simulink model "DUC"  (R2022a)
settings: Solver=VariableStepAuto  StartTime=0.0  StopTime=sample_period*512*300  RelTol=1e-3
InitFcn:
  | sample_period=1/400e6;
  | coeffs_AIE_scaling;
  | dds=75e6; % ddfs frequency
undefined symbols (not defined in the file or in its folder): None, S, vsva2197, xcvc1902
libraries: aieDSP x10, aieBasic x4, dspmlti4 x4, aieUtilities x2, vmcUtilities x1
settings Model: Creator=mmi  LastModifiedBy=robg
settings DebuggingCC: ParameterOverflowMsg=warning  UnconnectedInputMsg=warning  UnconnectedOutputMsg=warning  UnconnectedLineMsg=warning
settings HardwareCC: ProdBitPerPointer=32  ProdBitPerSizeT=32  ProdBitPerPtrDiffT=32  ProdLargestAtomicFloat=None  ProdIntDivRoundTo=Undefined  ProdEndianess=Unspecified  ProdWordSize=32  ProdHWDeviceType=ASIC/FPGA->ASIC/FPGA  TargetBitPerLong=64  TargetBitPerPointer=64  TargetBitPerSizeT=64  TargetBitPerPtrDiffT=64  TargetLongLongMode=on  TargetIntDivRoundTo=Zero  TargetEndianess=LittleEndian  TargetWordSize=64  TargetHWDeviceType=Custom Processor->MATLAB Host Computer  ProdEqTarget=off
settings RTWCC: DLArmComputeVersion=19.05

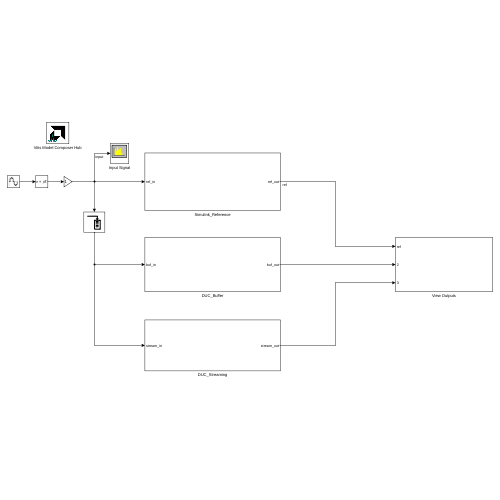
[thumbnail: Simulink's stored preview of the top-level diagram]
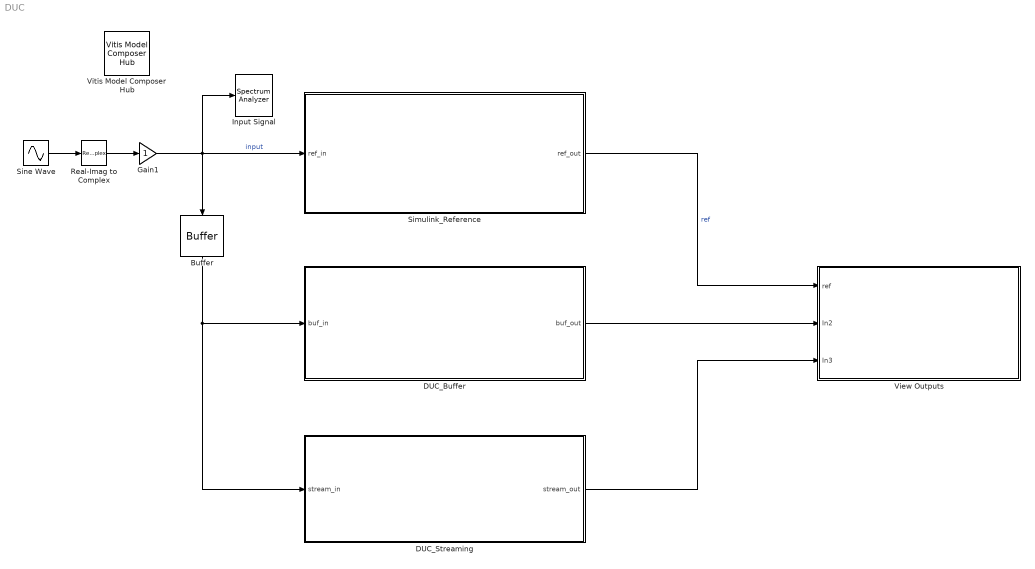
== system DUC ==
  Buffer : Buffer  N=32  OutputFrames=off
  DUC_Buffer : Subsystem
  DUC_Streaming : Subsystem
  Gain1 : Gain  OutDataTypeStr=fixdt(1,32,0)  RndMeth=Convergent
  Input Signal : SpectrumAnalyzer  DefaultConfigurationName=spbscopes.SpectrumAnalyzerBlockCfg
  Real-Imag to Complex : RealImagToComplex  Input=Real
  Simulink_Reference : Subsystem
  Sine Wave : Sin  Amplitude=1000  Frequency=2*pi*1e6  SampleTime=16*sample_period
  View Outputs : Subsystem
  Vitis Model Composer Hub : vmcUtilities/Vitis Model Composer Hub  Tag=genX  CodeGeneration=off  SubsystemName=DUC_Streaming  CompilationType=AIECompilation  ExportTypeV2=Graph Code  TargetDirectory=./duc_strm  exportDesign=off  analyzeDesign=on  validateDesignOnHw=off  ExportType=AI Engines  IpVendor=xilinx.com  IpLibrary=hls  IpVersion=1.0  IpHWLanguage=Verilog  AieCompilerOptions={}  AieSimulatorOptions={}  CreateTestbench=on  TestbenchStackSize=10  RunRtlSim=off  RunCSim=off  RunAieSim=on  AieSimTimeout=50000  RunAieSimProfiling=off  LaunchVitisAnalyzer=on  PlotOutput=off  RunX86Sim=off  X86SimTimeout=10  GenHwImage=off  GenLibadfXo=off  GenHwValidationCode=off  PlatformType=Not Specified  HwSystemType=Baremetal  HwValidationTarget=hw  ProjDevice=Versal VCK190 Evaluation Platform with New SD Level Shifter (xcvc1902-vsva2197-2MP-e-S)  ProjDevicePart=xcvc1902-vsva2197-2MP-e-S  AIEType=AIE  SamplePeriod=-1  ClockFrequency=200  DataPathParallelism=1  xilinxfamily=versalaicore  part=xcvc1902  speed=-2MP-e-S  package=vsva2197  directory=./netlist  testbench=off  incr_netlist=off  synthesis_tool=Vivado  clock_wrapper=Clock Enables  dbl_ovrd=According to Block Masks  dcm_input_clock_period=10  sysclk_period=sample_period  simulink_period=sample_period  eval_field=0  IPInfoJsonString="{\"AIESubsystem\":{\"SubsystemName\":\"DUC_Streaming\",\"TargetDirectory\":\"./duc_strm\",\"SubsystemDir\":\"./duc_strm/ip/DUC_Streaming\"},\"SubsystemTag\":\"AIENode\"}"  LogFileName=/group/xcoswmktg2/robg/git/vmc_examples/Vitis_Model_Composer/Examples/AIENGINE/DSPlib/DUC/duc_strm/model_composer.log  NThreads=4
  wires:
  Buffer/1 -> DUC_Streaming/1(stream_in), DUC_Buffer/1(buf_in)
  Sine Wave/1 -> Real-Imag to Complex/1
  Real-Imag to Complex/1 -> Gain1/1
  Gain1/1 -> Buffer/1, Input Signal/1, Simulink_Reference/1(ref_in)  "input"
  Simulink_Reference/1(ref_out) -> View Outputs/1(ref)  "ref"
  DUC_Buffer/1(buf_out) -> View Outputs/2(In2)
  DUC_Streaming/1(stream_out) -> View Outputs/3(In3)

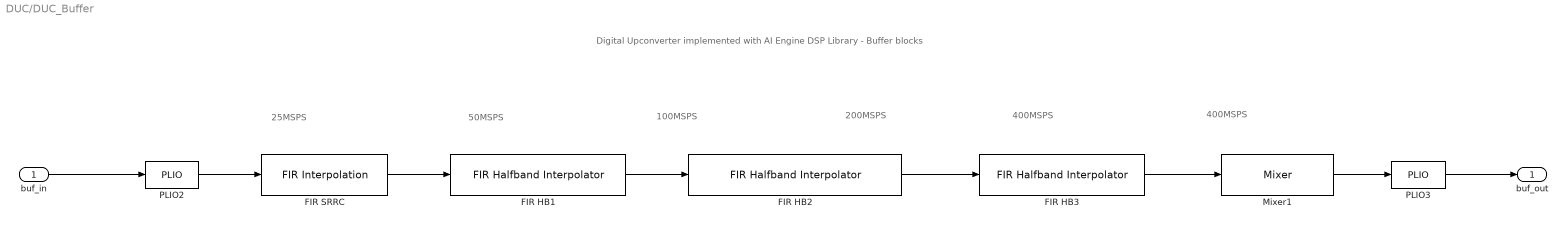
== system DUC/DUC_Buffer ==
  note: Digital Upconverter implemented with AI Engine DSP Library - Buffer blocks
  note: 25MSPS
  note: 400MSPS
  note: 100MSPS
  note: 400MSPS
  note: 50MSPS
  note: 200MSPS
  buf_in : Inport
  FIR HB1 : aieDSP/FIR Halfband Interpolator  data_type=cint32  coef_type=int32  use_coeff_reload=off  dual_ip=off  num_outputs=off  coeff=hb1_dsplib_coeff  fir_length=31  input_window_size=64  shift_val=17  rnd_mode=Round convergent to even  sat_mode=0-None  interp_poly=1  upshift_ct=0  casc_length=1  AIE_VARIANT=1  blockJsonConstraints=[]  blockJsonConstraintsInternal="{\"type\":\"constraint\",\"constraintType\":\"coreUtilization\",\"sid\":\"347:filter.m_firKernels[0]\",\"lhs\":{\"type\":\"runtimeRatio\",\"args\":{\"type\":\"kernel\",\"name\":\"dsplibDUC/AIE_DUC_Win/FIR HB1\",\"sid\":\"347:filter.m_firKernels[0]\"}},\"rhs\":{\"type\":\"evaluable\",\"expr\":\"0.2732\",\"value\":0.2732},\"equality\":true}"  spec=vmc_fir_interpolate_hb.json  SerializedMaskParamNames=[]  SerializedMaskParamValues=[]  SerializedMaskParamVisibilities=[]  block_type=FIR Halfband Interpolator  SerializedMaskParamDataypes=typename|typename|bool|bool|bool|coef_type|uint|uint|uint|uint|uint|uint|uint|uint|uint  SerializedMaskParamEnumStrArr=0|0|0|0|0|0|0|0|0|Floor,Ceiling,Round to positive infinity,Round to negative infinity,Round symmetrical to infinity,Round symmetrical to zero,Round convergent to even,Round convergent to odd|0-None,1-Asymmetric,3-Symmetric|0|0|0|0  SerializedMaskParamEnumValArr=0|0|0|0|0|0|0|0|0|0,1,2,3,4,5,6,7|0,1,3|0|0|0|0  SerializedMaskParamVectorArr=0|0|0|0|0|1|0|0|0|0|0|0|0|0|0
  FIR HB2 : aieDSP/FIR Halfband Interpolator  data_type=cint32  coef_type=int32  use_coeff_reload=off  dual_ip=off  num_outputs=off  coeff=hb2_dsplib_coeff  fir_length=31  input_window_size=128  shift_val=18  rnd_mode=Round convergent to even  sat_mode=0-None  interp_poly=1  upshift_ct=0  casc_length=1  AIE_VARIANT=1  blockJsonConstraints=[]  blockJsonConstraintsInternal="{\"type\":\"constraint\",\"constraintType\":\"coreUtilization\",\"sid\":\"348:filter.m_firKernels[0]\",\"lhs\":{\"type\":\"runtimeRatio\",\"args\":{\"type\":\"kernel\",\"name\":\"dsplibDUC/AIE_DUC_Win/FIR HB2\",\"sid\":\"348:filter.m_firKernels[0]\"}},\"rhs\":{\"type\":\"evaluable\",\"expr\":\"0.4057\",\"value\":0.4057},\"equality\":true}"  spec=vmc_fir_interpolate_hb.json  SerializedMaskParamNames=[]  SerializedMaskParamValues=[]  SerializedMaskParamVisibilities=[]  block_type=FIR Halfband Interpolator  SerializedMaskParamDataypes=typename|typename|bool|bool|bool|coef_type|uint|uint|uint|uint|uint|uint|uint|uint|uint  SerializedMaskParamEnumStrArr=0|0|0|0|0|0|0|0|0|Floor,Ceiling,Round to positive infinity,Round to negative infinity,Round symmetrical to infinity,Round symmetrical to zero,Round convergent to even,Round convergent to odd|0-None,1-Asymmetric,3-Symmetric|0|0|0|0  SerializedMaskParamEnumValArr=0|0|0|0|0|0|0|0|0|0,1,2,3,4,5,6,7|0,1,3|0|0|0|0  SerializedMaskParamVectorArr=0|0|0|0|0|1|0|0|0|0|0|0|0|0|0
  FIR HB3 : aieDSP/FIR Halfband Interpolator  data_type=cint32  coef_type=int32  use_coeff_reload=off  dual_ip=off  num_outputs=off  coeff=hb3_dsplib_coeff  fir_length=31  input_window_size=256  shift_val=16  rnd_mode=Round convergent to even  sat_mode=0-None  interp_poly=1  upshift_ct=0  casc_length=1  AIE_VARIANT=1  blockJsonConstraints=[]  blockJsonConstraintsInternal="{\"type\":\"constraint\",\"constraintType\":\"coreUtilization\",\"sid\":\"349:filter.m_firKernels[0]\",\"lhs\":{\"type\":\"runtimeRatio\",\"args\":{\"type\":\"kernel\",\"name\":\"dsplibDUC/AIE_DUC_Win/FIR HB3\",\"sid\":\"349:filter.m_firKernels[0]\"}},\"rhs\":{\"type\":\"evaluable\",\"expr\":\"0.8048\",\"value\":0.8048},\"equality\":true}"  spec=vmc_fir_interpolate_hb.json  SerializedMaskParamNames=[]  SerializedMaskParamValues=[]  SerializedMaskParamVisibilities=[]  block_type=FIR Halfband Interpolator  SerializedMaskParamDataypes=typename|typename|bool|bool|bool|coef_type|uint|uint|uint|uint|uint|uint|uint|uint|uint  SerializedMaskParamEnumStrArr=0|0|0|0|0|0|0|0|0|Floor,Ceiling,Round to positive infinity,Round to negative infinity,Round symmetrical to infinity,Round symmetrical to zero,Round convergent to even,Round convergent to odd|0-None,1-Asymmetric,3-Symmetric|0|0|0|0  SerializedMaskParamEnumValArr=0|0|0|0|0|0|0|0|0|0,1,2,3,4,5,6,7|0,1,3|0|0|0|0  SerializedMaskParamVectorArr=0|0|0|0|0|1|0|0|0|0|0|0|0|0|0
  FIR SRRC : aieDSP/FIR Interpolation  data_type=cint32  coef_type=int32  use_coeff_reload=off  num_outputs=off  coeff=srrc_coeff  fir_length=32  interpolate_factor=2  input_window_size=32  shift_val=12  rnd_mode=Round convergent to even  sat_mode=0-None  interp_poly=1  casc_length=1  AIE_VARIANT=1  blockJsonConstraints=[]  blockJsonConstraintsInternal="{\"type\":\"constraint\",\"constraintType\":\"coreUtilization\",\"sid\":\"350:filter.m_firKernels[0]\",\"lhs\":{\"type\":\"runtimeRatio\",\"args\":{\"type\":\"kernel\",\"name\":\"dsplibDUC/AIE_DUC_Win/FIR SRRC\",\"sid\":\"350:filter.m_firKernels[0]\"}},\"rhs\":{\"type\":\"evaluable\",\"expr\":\"0.5155\",\"value\":0.5155},\"equality\":true}"  spec=vmc_fir_interpolate_asym.json  SerializedMaskParamNames=[]  SerializedMaskParamValues=[]  SerializedMaskParamVisibilities=[]  block_type=FIR Interpolation  SerializedMaskParamDataypes=typename|typename|bool|bool|coef_type|uint|uint|uint|uint|uint|uint|uint|uint|uint  SerializedMaskParamEnumStrArr=0|0|0|0|0|0|0|0|0|Floor,Ceiling,Round to positive infinity,Round to negative infinity,Round symmetrical to infinity,Round symmetrical to zero,Round convergent to even,Round convergent to odd|0-None,1-Asymmetric,3-Symmetric|0|0|0  SerializedMaskParamEnumValArr=0|0|0|0|0|0|0|0|0|0,1,2,3,4,5,6,7|0,1,3|0|0|0  SerializedMaskParamVectorArr=0|0|0|0|1|0|0|0|0|0|0|0|0|0
  Mixer1 : aieDSP/Mixer  data_type=cint32  input_window_size=512  rnd_mode=Round to positive infinity  sat_mode=0-None  mixer_mode=Single Input Mode  USE_PHASE_RELOAD=off  phase_increment=805306368 % 75*2^32/400  AIE_VARIANT=1  blockJsonConstraints=[]  blockJsonConstraintsInternal=[]  spec=vmc_mixer.json  SerializedMaskParamNames=[]  SerializedMaskParamValues=[]  SerializedMaskParamVisibilities=[]  block_type=Mixer  SerializedMaskParamDataypes=typename|uint|uint|uint|uint|bool|uint|uint  SerializedMaskParamEnumStrArr=0|0|Floor,Ceiling,Round to positive infinity,Round to negative infinity,Round symmetrical to infinity,Round symmetrical to zero,Round convergent to even,Round convergent to odd|0-None,1-Asymmetric,3-Symmetric|Single Input Mode,Dual Input Mode|0|0|0  SerializedMaskParamEnumValArr=0|0|0,1,2,3,4,5,6,7|0,1,3|1,2|0|0|0  SerializedMaskParamVectorArr=0|0|0|0|0|0|0|0
  PLIO2 : aieBasic/PLIO  PlioWidth=64  PlioFreqSpec=on  PlioFreq=500  ColLocation=0  channel=0  blockJsonConstraints=[]  deprecateConstraints=0
  PLIO3 : aieBasic/PLIO  PlioWidth=64  PlioFreqSpec=on  PlioFreq=500  ColLocation=0  channel=0  blockJsonConstraints=[]  deprecateConstraints=0
  buf_out : Outport
  wires:
  PLIO2/1 -> FIR SRRC/1
  FIR HB1/1 -> FIR HB2/1
  FIR HB2/1 -> FIR HB3/1
  buf_in/1 -> PLIO2/1
  PLIO3/1 -> buf_out/1
  FIR HB3/1 -> Mixer1/1
  FIR SRRC/1 -> FIR HB1/1
  Mixer1/1 -> PLIO3/1

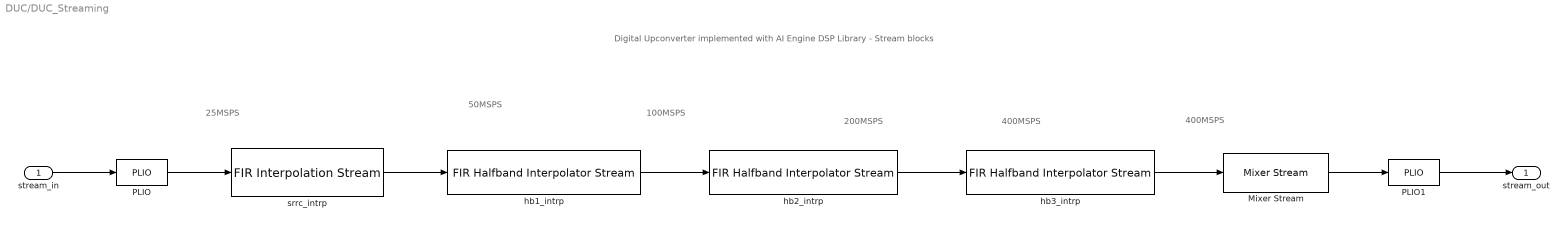
== system DUC/DUC_Streaming ==
  note: Digital Upconverter implemented with AI Engine DSP Library - Stream blocks
  note: 25MSPS
  note: 50MSPS
  note: 100MSPS
  note: 200MSPS
  note: 400MSPS
  note: 400MSPS
  stream_in : Inport
  Mixer Stream : aieDSP/Mixer Stream  data_type=cint32  input_window_size=512  mixer_mode=Single Input Mode  ssr=1  rnd_mode=Round to positive infinity  sat_mode=0-None  phase_increment=805306368 % 75*2^32/400  USE_PHASE_RELOAD=off  initial_phase_offset=0  AIE_VARIANT=1  blockJsonConstraints=[]  blockJsonConstraintsInternal=[]  spec=vmc_stream_mixer.json  SerializedMaskParamNames=[]  SerializedMaskParamValues=[]  SerializedMaskParamVisibilities=[]  block_type=Mixer Stream  SerializedMaskParamDataypes=typename|uint|uint|uint|uint|uint|uint|bool|uint|uint  SerializedMaskParamEnumStrArr=0|0|Single Input Mode,Dual Input Mode|0|Floor,Ceiling,Round to positive infinity,Round to negative infinity,Round symmetrical to infinity,Round symmetrical to zero,Round convergent to even,Round convergent to odd|0-None,1-Asymmetric,3-Symmetric|0|0|0|0  SerializedMaskParamEnumValArr=0|0|1,2|0|0,1,2,3,4,5,6,7|0,1,3|0|0|0|0  SerializedMaskParamVectorArr=0|0|0|0|0|0|0|0|0|0
  PLIO : aieBasic/PLIO  PlioWidth=64  PlioFreqSpec=on  PlioFreq=250  ColLocation=0  channel=0  blockJsonConstraints=[]  deprecateConstraints=0
  PLIO1 : aieBasic/PLIO  PlioWidth=64  PlioFreqSpec=on  PlioFreq=500  ColLocation=0  channel=0  blockJsonConstraints=[]  deprecateConstraints=0
  hb1_intrp : aieDSP/FIR Halfband Interpolator Stream  data_type=cint32  coef_type=int32  use_coeff_reload=off  dual_ip=off  num_outputs=off  coeff=hb1_dsplib_coeff  fir_length=31  input_window_size=64  shift_val=17  rnd_mode=Round convergent to even  sat_mode=0-None  ssr=1  interp_poly=1  upshift_ct=0  casc_length=2  AIE_VARIANT=1  blockJsonConstraints=[]  blockJsonConstraintsInternal=[]  spec=vmc_stream_fir_interpolate_hb.json  SerializedMaskParamNames=[]  SerializedMaskParamValues=[]  SerializedMaskParamVisibilities=[]  block_type=FIR Halfband Interpolator Stream  SerializedMaskParamDataypes=typename|typename|bool|bool|bool|coef_type|uint|uint|uint|uint|uint|uint|uint|uint|uint|uint  SerializedMaskParamEnumStrArr=0|0|0|0|0|0|0|0|0|Floor,Ceiling,Round to positive infinity,Round to negative infinity,Round symmetrical to infinity,Round symmetrical to zero,Round convergent to even,Round convergent to odd|0-None,1-Asymmetric,3-Symmetric|0|0|0|0|0  SerializedMaskParamEnumValArr=0|0|0|0|0|0|0|0|0|0,1,2,3,4,5,6,7|0,1,3|0|0|0|0|0  SerializedMaskParamVectorArr=0|0|0|0|0|1|0|0|0|0|0|0|0|0|0|0
  hb2_intrp : aieDSP/FIR Halfband Interpolator Stream  data_type=cint32  coef_type=int32  use_coeff_reload=off  dual_ip=off  num_outputs=off  coeff=hb2_dsplib_coeff  fir_length=31  input_window_size=128  shift_val=18  rnd_mode=Round convergent to even  sat_mode=0-None  ssr=1  interp_poly=1  upshift_ct=0  casc_length=1  AIE_VARIANT=1  blockJsonConstraints=[]  blockJsonConstraintsInternal=[]  spec=vmc_stream_fir_interpolate_hb.json  SerializedMaskParamNames=[]  SerializedMaskParamValues=[]  SerializedMaskParamVisibilities=[]  block_type=FIR Halfband Interpolator Stream  SerializedMaskParamDataypes=typename|typename|bool|bool|bool|coef_type|uint|uint|uint|uint|uint|uint|uint|uint|uint|uint  SerializedMaskParamEnumStrArr=0|0|0|0|0|0|0|0|0|Floor,Ceiling,Round to positive infinity,Round to negative infinity,Round symmetrical to infinity,Round symmetrical to zero,Round convergent to even,Round convergent to odd|0-None,1-Asymmetric,3-Symmetric|0|0|0|0|0  SerializedMaskParamEnumValArr=0|0|0|0|0|0|0|0|0|0,1,2,3,4,5,6,7|0,1,3|0|0|0|0|0  SerializedMaskParamVectorArr=0|0|0|0|0|1|0|0|0|0|0|0|0|0|0|0
  hb3_intrp : aieDSP/FIR Halfband Interpolator Stream  data_type=cint32  coef_type=int32  use_coeff_reload=off  dual_ip=off  num_outputs=off  coeff=hb3_dsplib_coeff  fir_length=31  input_window_size=256  shift_val=16  rnd_mode=Round convergent to even  sat_mode=0-None  ssr=1  interp_poly=1  upshift_ct=0  casc_length=1  AIE_VARIANT=1  blockJsonConstraints=[]  blockJsonConstraintsInternal=[]  spec=vmc_stream_fir_interpolate_hb.json  SerializedMaskParamNames=[]  SerializedMaskParamValues=[]  SerializedMaskParamVisibilities=[]  block_type=FIR Halfband Interpolator Stream  SerializedMaskParamDataypes=typename|typename|bool|bool|bool|coef_type|uint|uint|uint|uint|uint|uint|uint|uint|uint|uint  SerializedMaskParamEnumStrArr=0|0|0|0|0|0|0|0|0|Floor,Ceiling,Round to positive infinity,Round to negative infinity,Round symmetrical to infinity,Round symmetrical to zero,Round convergent to even,Round convergent to odd|0-None,1-Asymmetric,3-Symmetric|0|0|0|0|0  SerializedMaskParamEnumValArr=0|0|0|0|0|0|0|0|0|0,1,2,3,4,5,6,7|0,1,3|0|0|0|0|0  SerializedMaskParamVectorArr=0|0|0|0|0|1|0|0|0|0|0|0|0|0|0|0
  srrc_intrp : aieDSP/FIR Interpolation Stream  data_type=cint32  coef_type=int32  use_coeff_reload=off  dual_ip=off  num_outputs=off  coeff=srrc_coeff  fir_length=32  interpolate_factor=2  input_window_size=32  shift_val=12  rnd_mode=Round convergent to even  sat_mode=0-None  ssr=1  interp_poly=1  casc_length=4  AIE_VARIANT=1  blockJsonConstraints=[]  blockJsonConstraintsInternal="[{\"type\":\"constraint\",\"constraintType\":\"coreUtilization\",\"sid\":\"115:filter.m_firKernels[2]\",\"lhs\":{\"type\":\"runtimeRatio\",\"args\":{\"type\":\"kernel\",\"name\":\"dsplibDUC/AIE_DUC_stream/srrc_intrp\",\"sid\":\"115:filter.m_firKernels[2]\"}},\"rhs\":{\"type\":\"evaluable\",\"expr\":\"0.2\",\"value\":0.2},\"equality\":true},{\"type\":\"constraint\",\"constraintType\":\"coreUtilization\",\"sid\":\"115:filter.m_firKernels[3]\",\"lhs\":{\"type\":\"runtimeRatio\",\"args\":{\"type\":\"kernel\",\"name\":\"dsplibDUC/AIE_DUC_stream/srrc_intrp\",\"sid\":\"115:filter.m_firKernels[3]\"}},\"rhs\":{\"type\":\"evaluable\",\"expr\":\"0.2\",\"value\":0.2},\"equality\":true},{\"type\":\"constraint\",\"constraintType\":\"coreUtilization\",\"sid\":\"115:filter.m_firKernels[1]\",\"lhs\":{\"type\":\"runtimeRatio\",\"args\":{\"type\":\"kernel\",\"name\":\"dsplibDUC/AIE_DUC_stream/srrc_intrp\",\"sid\":\"115:filter.m_firKernels[1]\"}},\"rhs\":{\"type\":\"evaluable\",\"expr\":\"0.2\",\"value\":0.2},\"equality\":true},{\"type\":\"constraint\",\"constraintType\":\"coreUtilization\",\"sid\":\"115:filter.m_firKernels[0]\",\"lhs\":{\"type\":\"runtimeRatio\",\"args\":{\"type\":\"kernel\",\"name\":\"dsplibDUC/AIE_DUC_stream/srrc_intrp\",\"sid\":\"115:filter.m_firKernels[0]\"}},\"rhs\":{\"type\":\"evaluable\",\"expr\":\"0.2\",\"value\":0.2},\"equality\":true}]"  spec=vmc_stream_fir_interpolate_asym.json  SerializedMaskParamNames=[]  SerializedMaskParamValues=[]  SerializedMaskParamVisibilities=[]  block_type=FIR Interpolation Stream  SerializedMaskParamDataypes=typename|typename|bool|bool|bool|coef_type|uint|uint|uint|uint|uint|uint|uint|uint|uint|uint  SerializedMaskParamEnumStrArr=0|0|0|0|0|0|0|0|0|0|Floor,Ceiling,Round to positive infinity,Round to negative infinity,Round symmetrical to infinity,Round symmetrical to zero,Round convergent to even,Round convergent to odd|0-None,1-Asymmetric,3-Symmetric|0|0|0|0  SerializedMaskParamEnumValArr=0|0|0|0|0|0|0|0|0|0|0,1,2,3,4,5,6,7|0,1,3|0|0|0|0  SerializedMaskParamVectorArr=0|0|0|0|0|1|0|0|0|0|0|0|0|0|0|0
  stream_out : Outport
  wires:
  hb2_intrp/1 -> hb3_intrp/1
  stream_in/1 -> PLIO/1
  hb3_intrp/1 -> Mixer Stream/1
  PLIO1/1 -> stream_out/1
  PLIO/1 -> srrc_intrp/1
  Mixer Stream/1 -> PLIO1/1
  srrc_intrp/1 -> hb1_intrp/1
  hb1_intrp/1 -> hb2_intrp/1

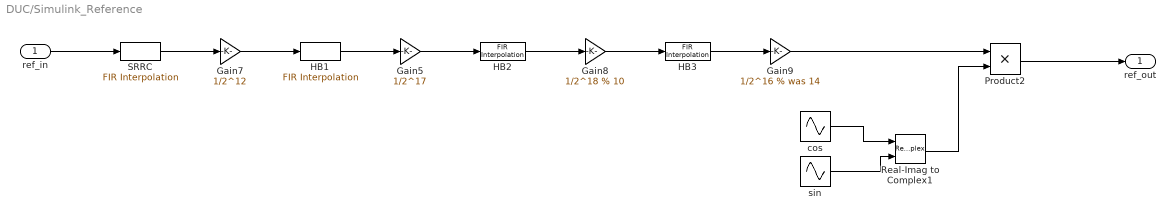
== system DUC/Simulink_Reference ==
  ref_in : Inport
  Gain5 : Gain  Gain=1/2^17  OutDataTypeStr=fixdt(1,32,0)  RndMeth=Convergent
  Gain7 : Gain  Gain=1/2^12  OutDataTypeStr=fixdt(1,32,0)  RndMeth=Convergent
  Gain8 : Gain  Gain=1/2^18 % 10  OutDataTypeStr=fixdt(1,32,0)  RndMeth=Convergent
  Gain9 : Gain  Gain=1/2^16 % was 14  OutDataTypeStr=fixdt(1,32,0)  RndMeth=Convergent
  HB1 : dspmlti4/FIR Interpolation  FilterSource=Dialog parameters  PrivateCoeffs=0  h=hb1_coeff  L=2  FilterObject=FINTERP  framing=Allow multirate processing  outputBufInitCond=0  roundingMode=Floor  overflowMode=off  firstCoeffMode=Specify word length  firstCoeffWordLength=18  firstCoeffFracLength=15  firstCoeffDataTypeStr=fixdt(1,18)  firstCoeffMin=[]  firstCoeffMax=[]  firstCoeffLastDataTypeStr=fixdt(1,18)  outputDataTypeStr=Inherit: Same as accumulator  outputMin=[]  outputMax=[]  outputLastDataTypeStr=Inherit: Same as accumulator
  HB2 : dspmlti4/FIR Interpolation  FilterSource=Dialog parameters  PrivateCoeffs=0  h=hb2_coeff  L=2  FilterObject=FINTERP  framing=Allow multirate processing  outputBufInitCond=0  roundingMode=Floor  overflowMode=off  firstCoeffMode=Specify word length  firstCoeffWordLength=18  firstCoeffFracLength=0  firstCoeffDataTypeStr=fixdt(1,18)  firstCoeffMin=[]  firstCoeffMax=[]  firstCoeffLastDataTypeStr=fixdt(1,18)  outputDataTypeStr=Inherit: Same as accumulator  outputMin=[]  outputMax=[]  outputLastDataTypeStr=Inherit: Same as accumulator
  HB3 : dspmlti4/FIR Interpolation  FilterSource=Dialog parameters  PrivateCoeffs=0  h=hb3_coeff  L=2  FilterObject=FINTERP  framing=Allow multirate processing  outputBufInitCond=0  roundingMode=Floor  overflowMode=off  firstCoeffMode=Specify word length  firstCoeffWordLength=18  firstCoeffFracLength=0  firstCoeffDataTypeStr=fixdt(1,18)  firstCoeffMin=[]  firstCoeffMax=[]  firstCoeffLastDataTypeStr=fixdt(1,18)  outputDataTypeStr=Inherit: Same as accumulator  outputMin=[]  outputMax=[]  outputLastDataTypeStr=Inherit: Same as accumulator
  Product2 : Product
  Real-Imag to Complex1 : RealImagToComplex
  SRRC : dspmlti4/FIR Interpolation  FilterSource=Dialog parameters  PrivateCoeffs=0  h=srrc_coeff  L=2  FilterObject=FINTERP  framing=Allow multirate processing  outputBufInitCond=0  roundingMode=Floor  overflowMode=off  firstCoeffMode=Specify word length  firstCoeffWordLength=18  firstCoeffFracLength=15  firstCoeffDataTypeStr=fixdt(1,18)  firstCoeffMin=[]  firstCoeffMax=[]  firstCoeffLastDataTypeStr=fixdt(1,18)  outputDataTypeStr=Inherit: Same as accumulator  outputMin=[]  outputMax=[]  outputLastDataTypeStr=Inherit: Same as accumulator
  cos : Sin  Frequency=dds*2*pi  Phase=pi/2  SampleTime=sample_period  VectorParams1D=off
  sin : Sin  Frequency=dds*2*pi  SampleTime=sample_period  VectorParams1D=off
  ref_out : Outport
  wires:
  sin/1 -> Real-Imag to Complex1/2
  Real-Imag to Complex1/1 -> Product2/2
  HB1/1 -> Gain5/1
  Gain7/1 -> HB1/1
  Gain8/1 -> HB3/1
  cos/1 -> Real-Imag to Complex1/1
  ref_in/1 -> SRRC/1
  HB3/1 -> Gain9/1
  HB2/1 -> Gain8/1
  Product2/1 -> ref_out/1
  SRRC/1 -> Gain7/1
  Gain5/1 -> HB2/1
  Gain9/1 -> Product2/1

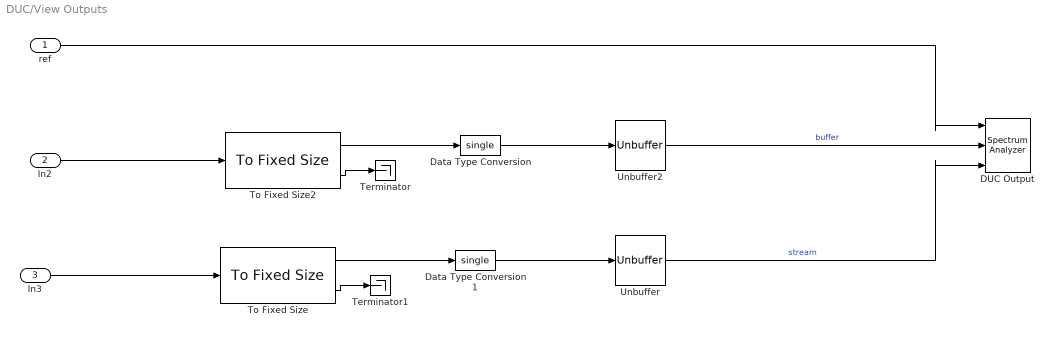
== system DUC/View Outputs ==
  ref : Inport
  In2 : Inport  Port=2
  In3 : Inport  Port=3
  DUC Output : SpectrumAnalyzer  NumInputPorts=3  DefaultConfigurationName=spbscopes.SpectrumAnalyzerBlockCfg
  Data Type Conversion : DataTypeConversion  OutDataTypeStr=single  SaturateOnIntegerOverflow=off  RndMeth=Floor
  Data Type Conversion1 : DataTypeConversion  OutDataTypeStr=single  SaturateOnIntegerOverflow=off  RndMeth=Floor
  Terminator : Terminator
  Terminator1 : Terminator
  To Fixed Size : aieUtilities/To Fixed Size  Mode=Produce a valid output signal  OutputSize=Inherit: Same as input  CopyMethod=Buffer samples to form output  HasStatusOutput=on
  To Fixed Size2 : aieUtilities/To Fixed Size  Mode=Produce a valid output signal  OutputSize=Inherit: Same as input  CopyMethod=Buffer samples to form output  HasStatusOutput=on
  Unbuffer : Unbuffer
  Unbuffer2 : Unbuffer
  wires:
  To Fixed Size/1 -> Data Type Conversion1/1
  Data Type Conversion/1 -> Unbuffer2/1
  In2/1 -> To Fixed Size2/1
  To Fixed Size/2 -> Terminator1/1
  Unbuffer2/1 -> DUC Output/2  "buffer"
  To Fixed Size2/1 -> Data Type Conversion/1
  Data Type Conversion1/1 -> Unbuffer/1
  Unbuffer/1 -> DUC Output/3  "stream"
  To Fixed Size2/2 -> Terminator/1
  In3/1 -> To Fixed Size/1
  ref/1 -> DUC Output/1
